simulink subsystem "Subsystem_PieroModel"  (R2023b)
settings: Solver=VariableStepAuto  StartTime=0.0  StopTime=10.0  RelTol=1e-3
settings Model: Creator=Alberto  LastModifiedBy=Alberto

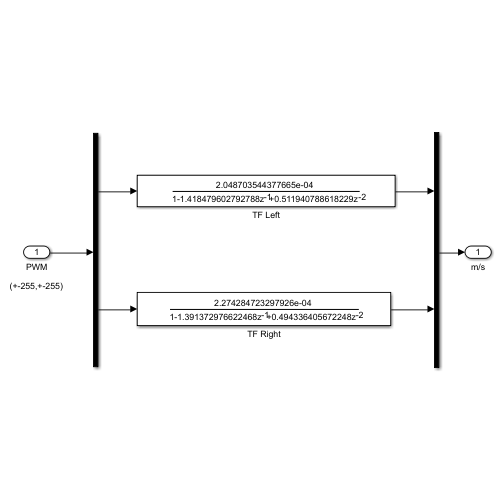
[thumbnail: Simulink's stored preview of the top-level diagram]
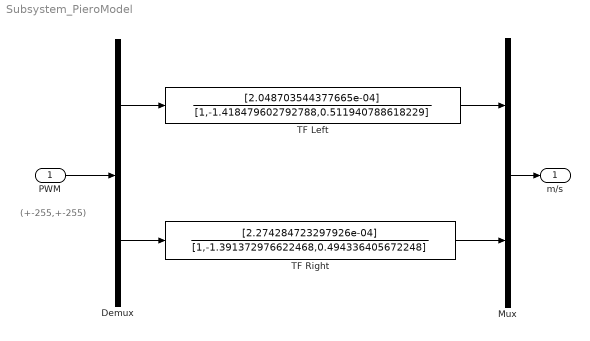
== system Subsystem_PieroModel ==
  note: (+-255,+-255)
  PWM : Inport
  Demux : Demux  Outputs=2
  Mux : Mux  Inputs=2
  TF Left : DiscreteFilter  Numerator=[2.048703544377665e-04]  Denominator=[1,-1.418479602792788,0.511940788618229]
  TF Right : DiscreteFilter  Numerator=[2.274284723297926e-04]  Denominator=[1,-1.391372976622468,0.494336405672248]
  m/s : Outport
  wires:
  PWM/1 -> Demux/1
  Mux/1 -> m/s/1
  Demux/1 -> TF Left/1
  TF Left/1 -> Mux/1
  Demux/2 -> TF Right/1
  TF Right/1 -> Mux/2
